simulink model "consensus_simple"  (R2025b)
settings: Solver=VariableStepAuto  StartTime=0.0  StopTime=10.0  RelTol=1e-3
undefined symbols (not defined in the file): L
settings Model: Creator=User  LastModifiedBy=User

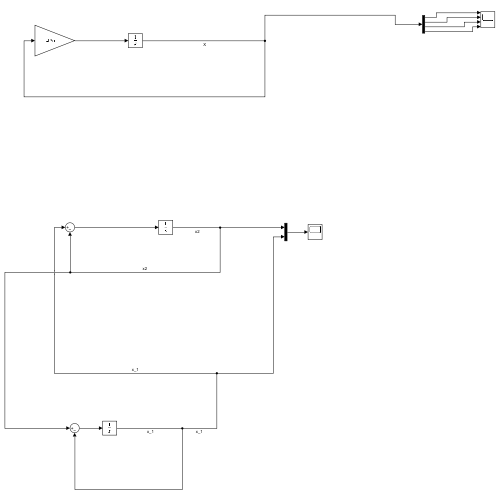
[thumbnail: Simulink's stored preview of the top-level diagram]
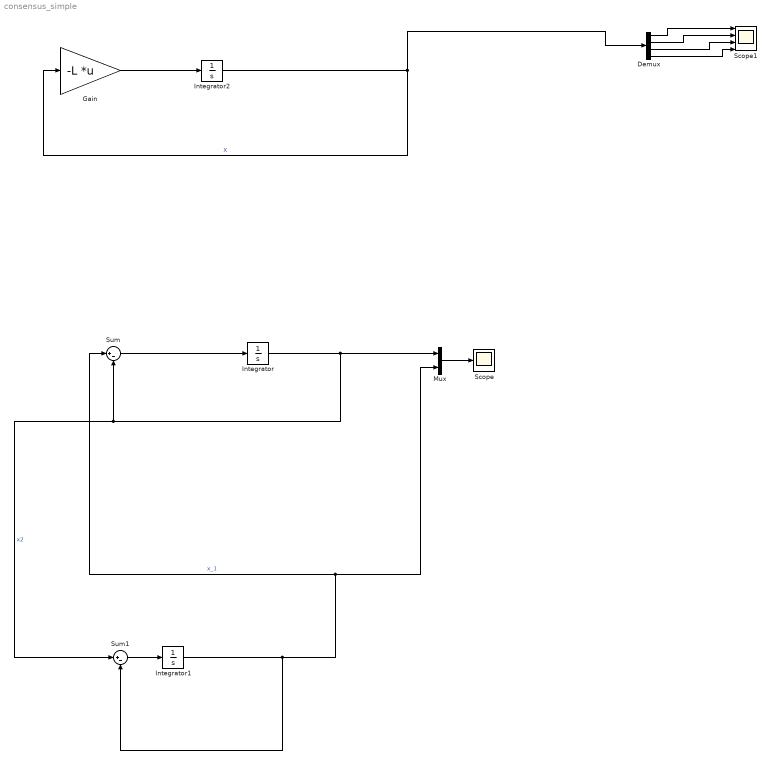
== system consensus_simple ==
  Demux : Demux
  Gain : Gain  Gain=-L  Multiplication=Matrix(K*u)
  Integrator : Integrator  InitialCondition=8
  Integrator1 : Integrator
  Integrator2 : Integrator  InitialCondition=[0;3;0;-3]
  Mux : Mux  Inputs=2
  Scope : Scope
      settings: ActiveDisplayYMinimum=-1  ActiveDisplayYMaximum=1
  Scope1 : Scope  NumInputPorts=4
      settings: ActiveDisplayYMinimum=-3.75  ActiveDisplayYMaximum=3.75
  Sum : Sum  Inputs=|+-
  Sum1 : Sum  Inputs=|+-
  wires:
  Integrator/1 -> Sum1/1, Sum/2, Mux/1  "x2"
  Sum/1 -> Integrator/1
  Integrator1/1 -> Mux/2, Sum/1, Sum1/2  "x_1"
  Sum1/1 -> Integrator1/1
  Mux/1 -> Scope/1
  Gain/1 -> Integrator2/1
  Integrator2/1 -> Demux/1, Gain/1  "X"
  Demux/1 -> Scope1/1
  Demux/3 -> Scope1/3
  Demux/4 -> Scope1/4
  Demux/2 -> Scope1/2
